simulink model "tanque"  (R2020a)
settings: Solver=VariableStepAuto  StartTime=0.0  StopTime=60  MaxStep=1e-2  RelTol=1e-3
undefined symbols (not defined in the file): h0, Kb, Kt
settings Model: Creator=a1  LastModifiedBy=a1

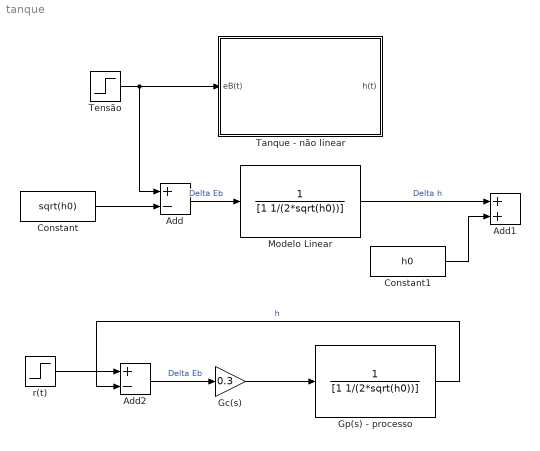
== system tanque ==
  Add : Sum  Inputs=+-
  Add1 : Sum
  Add2 : Sum  Inputs=+-
  Constant : Constant  Value=sqrt(h0)
  Constant1 : Constant  Value=h0
  Gc(s) : Gain  Gain=0.3
  Gp(s) - processo : TransferFcn  Denominator=[1 1/(2*sqrt(h0))]
  Modelo Linear : TransferFcn  Denominator=[1 1/(2*sqrt(h0))]
  Tanque - não linear : Subsystem
  Tensão : Step  Time=10  Before=sqrt(h0)  After=sqrt(1.1*h0)  SampleTime=0
  r(t) : Step  Time=10  SampleTime=0
  wires:
  Tensão/1 -> Add/1, Tanque - não linear/1(eB(t))
  Constant/1 -> Add/2
  Add/1 -> Modelo Linear/1  "Delta Eb"
  Modelo Linear/1 -> Add1/1  "Delta h"
  Constant1/1 -> Add1/2
  r(t)/1 -> Add2/1
  Gc(s)/1 -> Gp(s) - processo/1
  Add2/1 -> Gc(s)/1  "Delta Eb"
  Gp(s) - processo/1 -> Add2/2  "h"

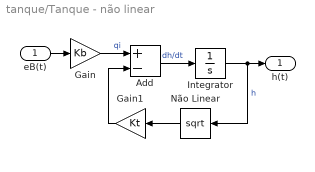
== system tanque/Tanque - não linear ==
  eB(t) : Inport
  Add : Sum  Inputs=+-
  Gain : Gain  Gain=Kb
  Gain1 : Gain  Gain=Kt
  Integrator : Integrator  InitialCondition=h0
  Não Linear : Sqrt  SaturateOnIntegerOverflow=on
  h(t) : Outport
  wires:
  eB(t)/1 -> Gain/1
  Integrator/1 -> h(t)/1, Não Linear/1  "h"
  Não Linear/1 -> Gain1/1
  Gain1/1 -> Add/2
  Gain/1 -> Add/1  "qi"
  Add/1 -> Integrator/1  "dh/dt"
